simulink model "Closed_Loop_Model"  (R2020a)
settings: Solver=VariableStepAuto  StartTime=0.0  StopTime=inf  RelTol=1e-3
libraries: vrlib x8, visionsinks x1
settings Model: Creator=Jeffrey  LastModifiedBy=Jeffrey

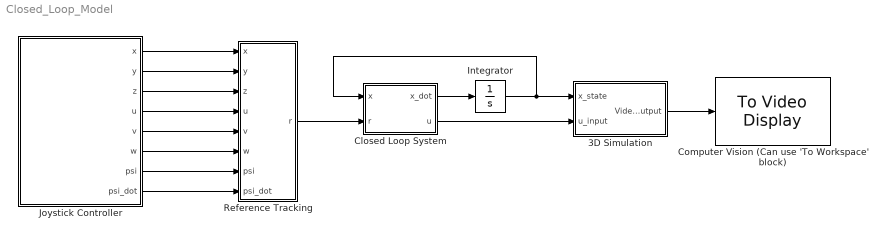
== system Closed_Loop_Model ==
  3D Simulation : Subsystem
  Closed Loop System : MATLAB Function  TreatAsAtomicUnit=on
  Computer Vision (Can use 'To Workspace' block) : visionsinks/To Video Display  windowSizeMode=Normal  openAtMdlStart=on  fullScreen=off  videoWindowX=536805376  videoWindowY=536805376  saveWindowSize=off  videoWindowWidth=640  videoWindowHeight=400  inputColorFormat=RGB  inputType=Obsolete  imagePorts=One multidimensional signal  OutputDevice=On-screen video monitor  dataOrg=Column-major  isWindowOpen=off
  Integrator : Integrator  InitialCondition=[0; 0; -1; 0; 0; 0; 0; 0; 0; 0; 0; 0]
  Joystick Controller : Subsystem
  Reference Tracking : MATLAB Function  TreatAsAtomicUnit=on
  wires:
  Integrator/1 -> 3D Simulation/1(x_state), Closed Loop System/1(x)
  Closed Loop System/1(x_dot) -> Integrator/1
  Reference Tracking/1(r) -> Closed Loop System/2(r)
  Joystick Controller/1(x) -> Reference Tracking/1(x)
  Joystick Controller/2(y) -> Reference Tracking/2(y)
  Joystick Controller/3(z) -> Reference Tracking/3(z)
  Joystick Controller/4(u) -> Reference Tracking/4(u)
  Joystick Controller/5(v) -> Reference Tracking/5(v)
  Joystick Controller/6(w) -> Reference Tracking/6(w)
  Joystick Controller/7(psi) -> Reference Tracking/7(psi)
  Joystick Controller/8(psi_dot) -> Reference Tracking/8(psi_dot)
  Closed Loop System/2(u) -> 3D Simulation/2(u_input)
  3D Simulation/1(Video Output) -> Computer Vision (Can use 'To Workspace' block)/1

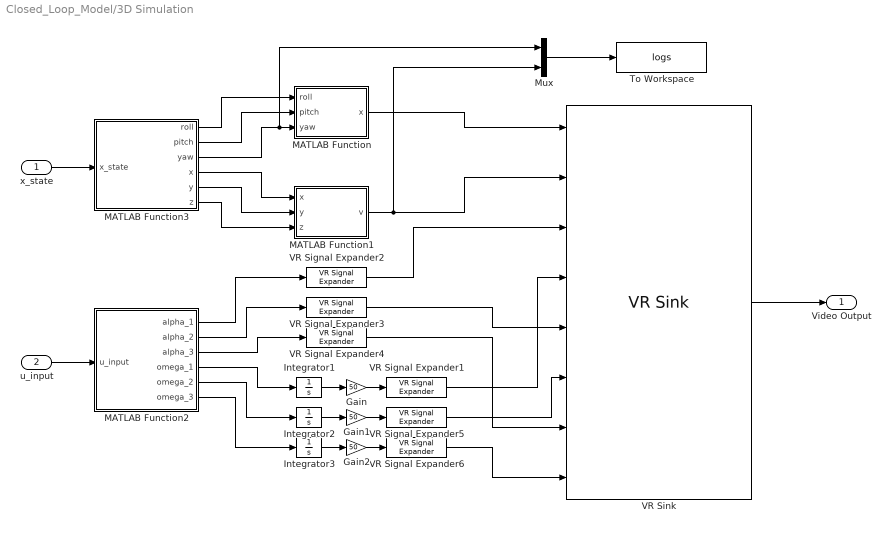
== system Closed_Loop_Model/3D Simulation ==
  x_state : Inport
  u_input : Inport  Port=2
  Gain : Gain  Gain=50
  Gain1 : Gain  Gain=50
  Gain2 : Gain  Gain=50
  Integrator1 : Integrator
  Integrator2 : Integrator
  Integrator3 : Integrator
  MATLAB Function : MATLAB Function  TreatAsAtomicUnit=on
  MATLAB Function1 : MATLAB Function  TreatAsAtomicUnit=on
  MATLAB Function2 : MATLAB Function  TreatAsAtomicUnit=on
  MATLAB Function3 : MATLAB Function  TreatAsAtomicUnit=on
  Mux : Mux  Inputs=2
  To Workspace : ToWorkspace  VariableName=logs  SampleTime=-1
      settings: Save2DSignal=2-D array (concatenate along first dimension)
  VR Signal Expander{1..6} (6 alike) : vrlib/VR Signal Expander  outwidth=4  outidx=[4]
  VR Sink : vrlib/VR Sink  InstantiateOnLoad=on  SampleTime=0.1  ViewEnable=on  RemoteChange=off  RemoteView=off  FieldsWritten=Airship.rotation.4.1.1.double#Airship.translation.3.1.1.double#Motor001.rotation.4.1.1.double#Prop001.rotation.4.1.1.double#Motor002.rotation.4.1.1.double#Prop002.rotation.4.1.1.double#Motor003.rotation.4.1.1.double#Prop003.rotation.4.1.1.double  WorldFileName=3DModel\3DModelTemplate.x3d  WorldDescription=Autonomous Airship  AutoView=on  VideoDimensions=[400 640]  AllowVariableSize=off  FigureProperties="{'Position', 'Name', 'Viewpoint', 'CameraBound', 'CameraDirection', 'CameraPosition', 'CameraUpVector', 'ZoomFactor', 'Antialiasing', 'Headlight', 'Lighting', 'NavPanel', 'Sound', 'StatusBar', 'Stereo3D', 'Stereo3DCameraOffset', 'Stereo3DHIT', 'ToolBar', 'Textures', 'Transparency', 'Triad', 'Wireframe', 'NavZones', 'NavMode', 'NavSpeed', 'CaptureFileFormat', 'CaptureFileName', 'Record2DCompressMethod', 'Record2DCompressQuality', 'Record2D', 'Record2DFileName', 'Record2DFPS'; [5.0000000000000000e+00   9.2000000000000000e+01   5.7600000000000000e+02   3.5000000000000000e+02], 'Autonomous Airship', 'SensorCam ', 'on', [0.0000000000000000e+00   0.0000000000000000e+00  -1.0000000000000000e+00], [0.0000000000000000e+00   0.0000000000000000e+00   0.0000000000000000e+00], [0.0000000000000000e+00   1.0000000000000000e+00   0.0000000000000000e+00], [1.0000000000000000e+00], 'on', 'on', 'on', 'halfbar', 'on', 'on', 'off', [1.0000000149011612e-01], [0.0000000000000000e+00], 'on', 'on', 'on', 'none', 'off', 'off', 'fly', 'normal', 'tif', '%f_anim_%n.tif', 'auto', [7.5000000000000000e+01], 'off', '%f_anim_%n.avi', 'auto'; [5.8600000000000000e+02   6.0000000000000000e+01   6.4000000000000000e+02   4.0000000000000000e+02], 'Autonomous Airship', 'SensorCam ', 'on', [0.0000000000000000e+00   0.0000000000000000e+00  -1.0000000000000000e+00], [0.0000000000000000e+00   0.0000000000000000e+00   0.0000000000000000e+00], [0.0000000000000000e+00   1.0000000000000000e+00   0.0000000000000000e+00], [1.0000000000000000e+00], 'on', 'on', 'on', 'none', 'on', 'off', 'off', [1.0000000149011612e-01], [0.0000000000000000e+00], 'off', 'on', 'on', 'none', 'off', 'off', 'fly', 'normal', 'tif', '%f_anim_%n.tif', 'auto', [7.5000000000000000e+01], 'off', '***video***', 'auto'}"
  Video Output : Outport
  wires:
  MATLAB Function3/5(y) -> MATLAB Function1/2(y)
  x_state/1 -> MATLAB Function3/1(x_state)
  VR Signal Expander6/1 -> VR Sink/8
  MATLAB Function/1(x) -> VR Sink/1
  VR Signal Expander3/1 -> VR Sink/5
  MATLAB Function3/4(x) -> MATLAB Function1/1(x)
  MATLAB Function2/2(alpha_2) -> VR Signal Expander3/1
  MATLAB Function2/3(alpha_3) -> VR Signal Expander4/1
  MATLAB Function2/1(alpha_1) -> VR Signal Expander2/1
  MATLAB Function3/1(roll) -> MATLAB Function/1(roll)
  VR Signal Expander5/1 -> VR Sink/6
  MATLAB Function2/5(omega_2) -> Integrator2/1
  Gain2/1 -> VR Signal Expander6/1
  Gain/1 -> VR Signal Expander1/1
  MATLAB Function3/6(z) -> MATLAB Function1/3(z)
  Gain1/1 -> VR Signal Expander5/1
  Integrator1/1 -> Gain/1
  MATLAB Function3/2(pitch) -> MATLAB Function/2(pitch)
  Integrator2/1 -> Gain1/1
  Integrator3/1 -> Gain2/1
  MATLAB Function3/3(yaw) -> Mux/1, MATLAB Function/3(yaw)
  VR Signal Expander2/1 -> VR Sink/3
  VR Signal Expander1/1 -> VR Sink/4
  VR Signal Expander4/1 -> VR Sink/7
  MATLAB Function2/6(omega_3) -> Integrator3/1
  MATLAB Function1/1(v) -> Mux/2, VR Sink/2
  MATLAB Function2/4(omega_1) -> Integrator1/1
  u_input/1 -> MATLAB Function2/1(u_input)
  Mux/1 -> To Workspace/1
  VR Sink/1 -> Video Output/1

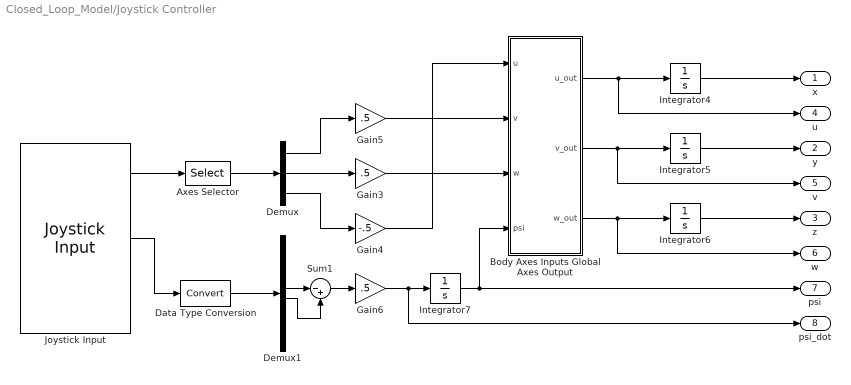
== system Closed_Loop_Model/Joystick Controller ==
  Axes Selector : Selector  InputPortWidth=5  IndexOptions=Index vector (dialog)  Indices=[1 3 2]  OutputSizes=1
      settings: AttributesFormatString=(Joystick - dependent)
  Body Axes Inputs Global Axes Output : MATLAB Function  TreatAsAtomicUnit=on
  Data Type Conversion : DataTypeConversion
  Demux : Demux  Outputs=3
  Demux1 : Demux  Outputs=10
  Gain3 : Gain  Gain=.5
  Gain4 : Gain  Gain=-.5
  Gain5 : Gain  Gain=.5
  Gain6 : Gain  Gain=.5
  Integrator4 : Integrator
  Integrator5 : Integrator
  Integrator6 : Integrator  InitialCondition=-1
  Integrator7 : Integrator
  Joystick Input : vrlib/Joystick Input  joyid=1  adjustports=on  forcefeed=off
  Sum1 : Sum  Inputs=|-+
  x : Outport
  y : Outport  Port=2
  z : Outport  Port=3
  u : Outport  Port=4
  v : Outport  Port=5
  w : Outport  Port=6
  psi : Outport  Port=7
  psi_dot : Outport  Port=8
  wires:
  Gain3/1 -> Body Axes Inputs Global Axes Output/3(w)
  Body Axes Inputs Global Axes Output/3(w_out) -> w/1, Integrator6/1
  Demux/2 -> Gain3/1
  Gain5/1 -> Body Axes Inputs Global Axes Output/2(v)
  Body Axes Inputs Global Axes Output/1(u_out) -> u/1, Integrator4/1
  Joystick Input/1 -> Axes Selector/1
  Axes Selector/1 -> Demux/1
  Joystick Input/2 -> Data Type Conversion/1
  Demux1/5 -> Sum1/1
  Demux/3 -> Gain4/1
  Gain4/1 -> Body Axes Inputs Global Axes Output/1(u)
  Demux/1 -> Gain5/1
  Sum1/1 -> Gain6/1
  Data Type Conversion/1 -> Demux1/1
  Demux1/6 -> Sum1/2
  Integrator5/1 -> y/1
  Body Axes Inputs Global Axes Output/2(v_out) -> v/1, Integrator5/1
  Integrator6/1 -> z/1
  Integrator4/1 -> x/1
  Integrator7/1 -> Body Axes Inputs Global Axes Output/4(psi), psi/1
  Gain6/1 -> psi_dot/1, Integrator7/1

== matlab function Closed_Loop_Model/3D Simulation/MATLAB Function1 ==
  data: x input; v output; y input; z input
function v = fcn(x,y,z)

v = [x , -z, y];

== matlab function Closed_Loop_Model/3D Simulation/MATLAB Function ==
  data: roll input; x output; pitch input; yaw input
function x = fcn(roll,pitch,yaw) %local pitch and roll
a = -roll;
b = -pitch;
c = yaw;

T_roll = [ 1, 0      , 0    ;
         0, cos(a) , sin(a) ;
         0, -sin(a), cos(a) ];
     
T_pitch = [cos(b),0,-sin(b) ;
        0     ,1,0       ;
        sin(b),0,cos(b)  ];
    
T_yaw = [cos(c) ,sin(c),0;
        -sin(c),cos(c),0;
        0      ,0     ,1];


T_BE = T_roll * T_pitch * T_yaw;
        
        
v = rotationMatrixToVector (T_BE^-1);

x = [v(1),v(3),v(2), norm(v)];

== matlab function Closed_Loop_Model/Reference Tracking ==
  data: x input; y input; z input; r output; u input; v input; w input; psi input; psi_dot input
function r = fcn(x,y,z,u,v,w,psi,psi_dot)

r = zeros(12,1);
% reference output
r(1) = x;
r(2) = y;
r(3) = z;
r(4) = u;
r(5) = v;
r(6) = w;
r(9) = psi;
r(12) = psi_dot;

== matlab function Closed_Loop_Model/3D Simulation/MATLAB Function3 ==
  data: roll output; pitch output; yaw output; x output; x_state input; y output; z output
function [roll,pitch,yaw,x,y,z] = fcn(x_state)

x = x_state(1);
y = x_state(2);
z = x_state(3);
roll = x_state(7);
pitch = x_state(8);
yaw = x_state(9);

== matlab function Closed_Loop_Model/3D Simulation/MATLAB Function2 ==
  data: alpha_1 output; alpha_2 output; alpha_3 output; omega_1 output; u_input input; omega_2 output; omega_3 output
function [alpha_1,alpha_2,alpha_3,omega_1,omega_2,omega_3] = fcn(u_input)

omega_1 = u_input(1);
omega_2 = u_input(2);
omega_3 = u_input(3);
alpha_1 = u_input(4);
alpha_2 = u_input(5);
alpha_3 = u_input(6);

== matlab function Closed_Loop_Model/Closed Loop System ==
  data: x input; x_dot output; r input; u output
function [x_dot,u] = fcn(x,r)
A = [0,0,0,1,0,0,0,0,0,0,0,0;0,0,0,0,1,0,0,0,0,0,0,0;0,0,0,0,0,1,0,0,0,0,0,0;0,0,0,0,0,0,0,-15,0,0,0,0;0,0,0,0,0,0,15,0,0,0,0,0;0,0,0,0,0,0,0,0,0,0,0,0;0,0,0,0,0,0,0,0,0,1,0,0;0,0,0,0,0,0,0,0,0,0,1,0;0,0,0,0,0,0,0,0,0,0,0,1;0,0,0,0,0,0,0,0,0,0,0,0;0,0,0,0,0,0,0,0,0,0,0,0;0,0,0,0,0,0,0,0,0,0,0,0];
B = [0,0,0,0,0,0;0,0,0,0,0,0;0,0,0,0,0,0;0,0,0,0,-4.33012701892219,4.33012701892219;0,0,0,5,-2.50000000000000,-2.50000000000000;-2,-2,-2,0,0,0;0,0,0,0,0,0;0,0,0,0,0,0;0,0,0,0,0,0;-0.625000000000000,0.998797632095823,-2.24879763209582,0.625000000000000,-8.48457346706593,5.04707346706593;1.80000000000000,0.900000000000000,0.900000000000000,7.50000000000000,-2.45096189432334,-5.04903810567666;-3.12500000000000,-2.80024047358084,-3.44975952641916,-4.37500000000000,-6.19691469341319,-3.49058530658681];
C = [8.99321605918731e-06,0,0,0,0,0,0,0,0,0,0,0;2.21564316353217e-19,8.99321605918742e-06,0,0,0,0,0,0,0,0,0,0;0,0,1,0,0,0,0,0,0,0,0,0;0,0,0,0.577350269189626,0.577350269189626,0.577350269189626,0,0,0,0,0,0;0,0,0,0,0,0,0,0,1,0,0,0;0,0,0,0,0,0,0,0,0,1,0,0;0,0,0,0,0,0,0,0,0,0,1,0;0,0,0,0,0,0,0,0,0,0,0,1];
D = [0,0,0,0,0,0;0,0,0,0,0,0;0,0,0,0,0,0;0,0,0,0,0,0;0,0,0,0,0,0;0,0,0,0,0,0;0,0,0,0,0,0;0,0,0,0,0,0];
K = [0.380455119485790,-1.60473285652832,-1.12796857058892,0.289082140016510,-1.96561152004540,-1.15381789835499,-5.60621429606471,2.88198241763627,-0.708277049069693,-0.0937550261943210,1.73655880446676,-0.728851704449303;-2.06549798801362,0.260161640764039,-1.96890858983730,-2.48406999114913,0.654397243163373,-2.31092222072699,7.72217160686784,6.15519804931563,-0.991201106392443,2.03196115028159,-0.430544586586357,-1.03710975933916;1.75196931557469,0.207062038526088,-1.57038720296227,2.07323261825993,0.0552336262162533,-1.64809695299470,-3.89689686633193,-4.69451688881825,-0.581454241433071,-1.81257556785601,0.258997650536400,-0.544156321772417;-0.607862402957131,1.65725153205730,0.894256287022723,-0.935070223207319,1.88026961997373,0.938683038624062,4.23231523319431,6.86092468228712,-1.66621413962186,1.08911146585114,1.85323226518509,-1.77552173278074;-0.368495229101924,-2.00405890819835,1.25622876243858,-0.272772810912930,-2.72146314509805,1.62450419795726,-13.3581530390366,-1.28083963630737,-1.61781508812281,-2.63200518028557,0.596292580704891,-1.67961878885800;1.41925686401502,0.742656679778377,0.0846456788220318,1.71555896650171,1.22107603751127,-0.00154406643539617,8.71836743904115,-6.89975405041296,-1.66858614855014,1.38016714215546,-2.77908379315661,-1.70580394002119];

u = K*(r-x);
x_dot = A*x+B*u;
%y=C*x

== matlab function Closed_Loop_Model/Joystick Controller/Body Axes Inputs Global Axes Output ==
  data: u input; u_out output; v input; w input; v_out output; w_out output; psi input
function [u_out,v_out,w_out] = fcn(u, v, w, psi)

%rotating uvw vector (assume input u v w in body frame)
a=0; b=0; c=psi;
T_roll = [ 1, 0      , 0    ;
         0, cos(a) , sin(a) ;
         0, -sin(a), cos(a) ];
     
T_pitch = [cos(b),0,-sin(b) ;
        0     ,1,0       ;
        sin(b),0,cos(b)  ];
    
T_yaw = [cos(c) ,sin(c),0;
        -sin(c),cos(c),0;
        0      ,0     ,1];

T_BE = T_roll * T_pitch * T_yaw;

v_e = T_BE^-1 * [u;v;w];

u_out = v_e(1);
v_out = v_e(2);
w_out = v_e(3);
